simulink model "full_loop"  (R2020a)
settings: Solver=FixedStepAuto  StartTime=0.0  StopTime=200  FixedStep=.005  RelTol=1e-3
model workspace (MAT data in the model file):
  SL_ROS_VariableLengthArrays_MaxSizes.CommonInfo.ArrayTruncateAction = 'EmitWarning'
  SL_ROS_VariableLengthArrays_MaxSizes.MsgTypeMap = containers.Map
  SL_ROS_VariableLengthArrays_MaxSizes.MsgTypeMap.serialization.keys = {}
  SL_ROS_VariableLengthArrays_MaxSizes.MsgTypeMap.serialization.values = {}
  SL_ROS_VariableLengthArrays_MaxSizes.MsgTypeMap.serialization.uniformity = 0
  SL_ROS_VariableLengthArrays_MaxSizes.MsgTypeMap.serialization.keyType = 'char'
  SL_ROS_VariableLengthArrays_MaxSizes.MsgTypeMap.serialization.valueType = 'any'
undefined symbols (not defined in the file): cf, gazeboStep, InitAUVPlant, InitController, modelName, referenceFrame, telemetryStep, trajec
libraries: robotlib x8
settings Model: SimulationMode=accelerator  PauseTimes=1000  Creator=Lamarre  LastModifiedBy=alexemdesgagne
settings OptimizationCC: EnhancedBackFolding=on  PassReuseOutputArgsAs=Individual arguments  ZeroExternalMemoryAtStartup=off  ZeroInternalMemoryAtStartup=off  MaxStackSize=64  OptimizeBlockOrder=speed  DifferentSizesBufferReuse=on  OptimizationCustomize=off  EfficientTunableParamExpr=on
settings DebuggingCC: ParameterTunabilityLossMsg=error
settings HardwareCC: ProdBitPerPointer=32  ProdBitPerSizeT=32  ProdBitPerPtrDiffT=32  ProdLargestAtomicInteger=Long  ProdWordSize=32  ProdHWDeviceType=ARM Compatible->ARM 8
settings SFSimCC: MATLABDynamicMemAlloc=off
settings RTWCC: SystemTargetFile=ert.tlc  HardwareBoard=Robot Operating System (ROS)  TemplateMakefile=ert_default_tmf  Toolchain=Catkin  BuildConfiguration=Faster Runs  TargetLang=C++
settings CodeAppCC: ForceParamTrailComments=on  IgnoreCustomStorageClasses=off  OperatorAnnotations=on  SimulinkDataObjDesc=on  SFDataObjDesc=on  InsertBlockDesc=on
settings ERTTargetCC: MultiInstanceERTCode=on  CodeInterfacePackaging=C++ class  SupportContinuousTime=on  SupportVariableSizeSignals=on  RootIOFormat=Structure reference

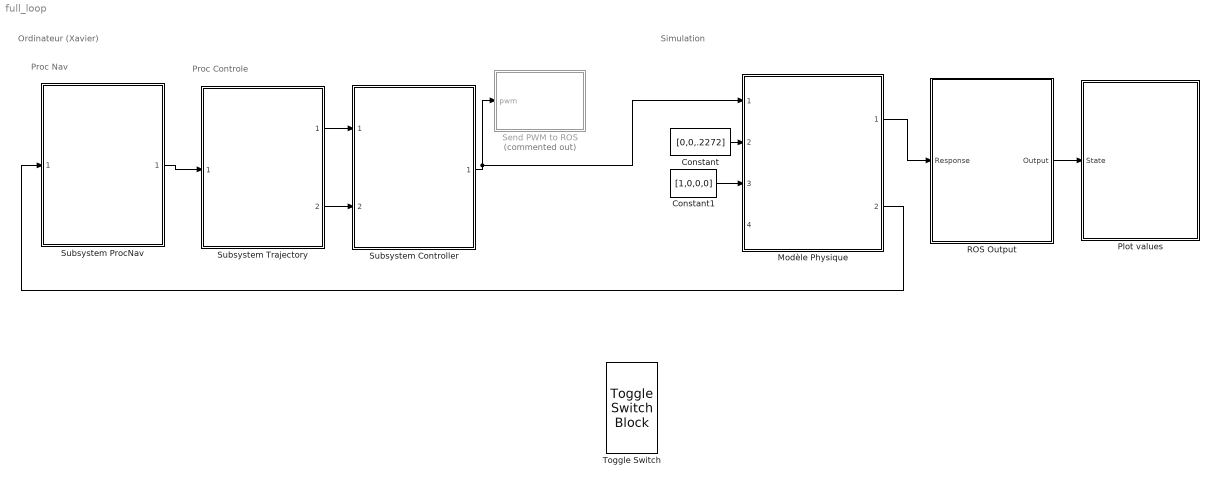
== system full_loop ==
  note: Simulation
  note: Proc Nav
  note: Proc Controle
  note: Ordinateur (Xavier)
  Constant : Constant  Value=[0,0,.2272]
  Constant1 : Constant  Value=[1,0,0,0]
  Modèle Physique : Subsystem  InitFcn=InitAUVPlant;  ReferencedSubsystem=AUVPlant
  Plot values : Subsystem
  ROS Output : Subsystem
  Send PWM to ROS : Subsystem  Commented=on
  Subsystem Controller : Subsystem  InitFcn=InitController;  ReferencedSubsystem=Controller
  Subsystem ProcNav : Subsystem  ReferencedSubsystem=ProcNav
  Subsystem Trajectory : Subsystem  InitFcn=trajec;  ReferencedSubsystem=Trajectory
  Toggle Switch : ToggleSwitchBlock
      settings: Values={{'Off', 'On'}, [0 1]}
  wires:
  Subsystem ProcNav/1 -> Subsystem Trajectory/1
  Subsystem Trajectory/1 -> Subsystem Controller/1
  Subsystem Controller/1 -> Modèle Physique/1, Send PWM to ROS/1(pwm)
  Modèle Physique/1 -> ROS Output/1(Response)
  Modèle Physique/2 -> Subsystem ProcNav/1
  Constant/1 -> Modèle Physique/2
  Constant1/1 -> Modèle Physique/3
  ROS Output/1(Output) -> Plot values/1(State)
  Subsystem Trajectory/2 -> Subsystem Controller/2

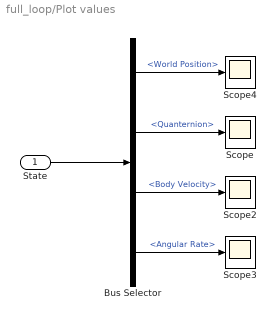
== system full_loop/Plot values ==
  State : Inport
  Bus Selector : BusSelector  OutputSignals=World Position,Quanternion,Body Velocity,Angular Rate
  Scope{,2..4} (4 alike) : Scope
  wires:
  Bus Selector/4 -> Scope3/1  "<Angular Rate>"
  State/1 -> Bus Selector/1
  Bus Selector/2 -> Scope/1  "<Quanternion>"
  Bus Selector/3 -> Scope2/1  "<Body Velocity>"
  Bus Selector/1 -> Scope4/1  "<World Position>"

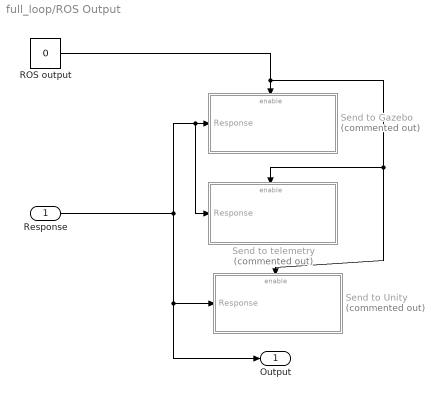
== system full_loop/ROS Output ==
  Response : Inport
  ROS output : Constant  Value=0
  Send to Gazebo : Subsystem  Commented=on  InitFcn=|
      | cf = ConfigAUV8();
      | 
      | % Parametres Messages ROS
      |     Duration = 229;
      |     gazeboStep=1/50;
      |     telemetryStep=1/30;
      |     referenceFrame = cf.referenceFrame;
      |     modelName = cf.modelName;
  Send to Unity : Subsystem  Commented=on  InitFcn=|
      | cf = ConfigAUV8();
      | 
      | % Parametres Messages ROS
      |     Duration = 229;
      |     gazeboStep=1/50;
      |     telemetryStep=1/30;
      |     referenceFrame = cf.referenceFrame;
      |     modelName = cf.modelName;
  Send to telemetry : Subsystem  Commented=on
  Output : Outport
  wires:
  Response/1 -> Send to telemetry/1(Response), Send to Gazebo/1(Response), Send to Unity/1(Response), Output/1
  ROS output/1 -> Send to Gazebo/Enable, Send to telemetry/Enable, Send to Unity/Enable

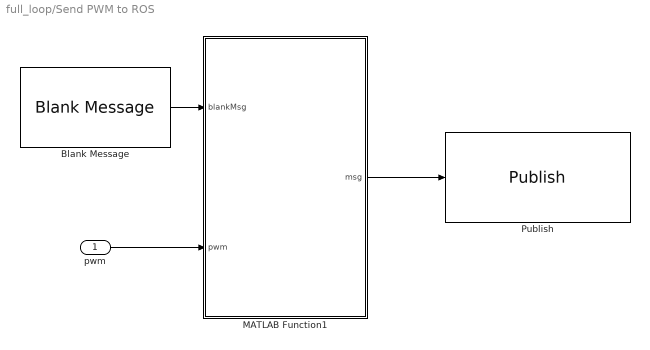
== system full_loop/Send PWM to ROS ==
  pwm : Inport
  Blank Message : robotlib/Blank Message  messageClass=Message  entityType=sonia_common/ThrusterPwm  messageType=sonia_common/ThrusterPwm  SampleTime=inf
  MATLAB Function1 : MATLAB Function  TreatAsAtomicUnit=on
  Publish : robotlib/Publish  topicSource=Specify your own  topic=/provider_thruster/thruster_pwm  messageType=sonia_common/ThrusterPwm  messageQueueLength=1
  wires:
  MATLAB Function1/1(msg) -> Publish/1
  Blank Message/1 -> MATLAB Function1/1(blankMsg)
  pwm/1 -> MATLAB Function1/2(pwm)

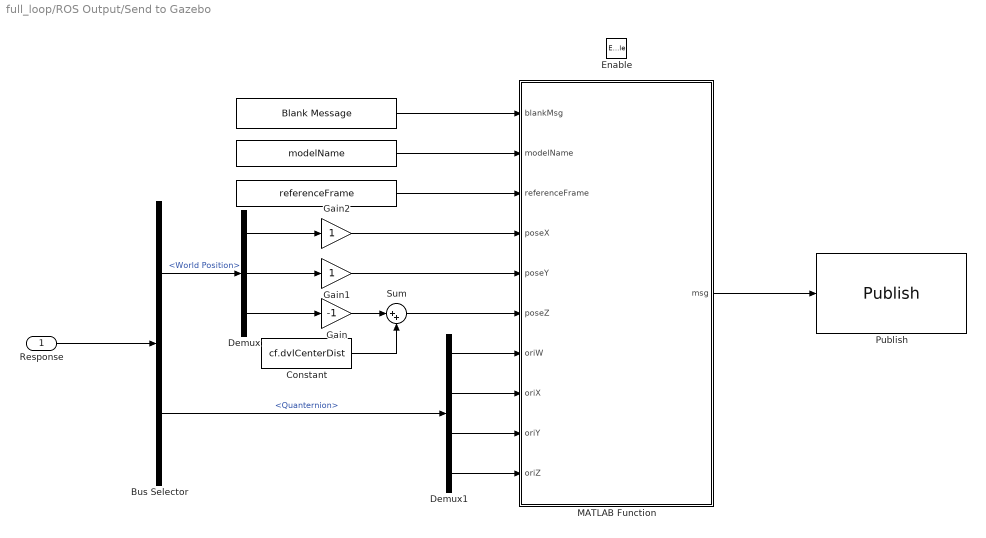
== system full_loop/ROS Output/Send to Gazebo ==
  Response : Inport
  Enable : EnablePort
  " " : Constant  Value=modelName  VectorParams1D=off
  "  " : Constant  Value=referenceFrame
  "   " : robotlib/Blank Message  messageClass=Message  entityType=gazebo_msgs/ModelState  messageType=gazebo_msgs/ModelState  SampleTime=1/50
  Bus Selector : BusSelector  OutputSignals=World Position,Quanternion
  Constant : Constant  Value=cf.dvlCenterDist
  Demux : Demux  Outputs=3
  Demux1 : Demux
  Gain : Gain  Gain=-1
  Gain1 : Gain
  Gain2 : Gain
  MATLAB Function : MATLAB Function  TreatAsAtomicUnit=on  SystemSampleTime=gazeboStep
  Publish : robotlib/Publish  topicSource=Select from ROS network  topic=/gazebo/set_model_state  messageType=gazebo_msgs/ModelState  messageQueueLength=1
      link override SinkBlock: ROSTopic=/gazebo/set_model_state  ROSMessageType=gazebo_msgs/ModelState  SLBusName=SL_Bus_plant_gazebo_msgs_ModelState  ModelName=plant  BlockId=Pub_plant_206
  Sum : Sum  Inputs=|++
  wires:
  Bus Selector/1 -> Demux/1  "<World Position>"
  Demux/1 -> Gain2/1
  Demux/2 -> Gain1/1
  Demux/3 -> Gain/1
  "   "/1 -> MATLAB Function/1(blankMsg)
  "  "/1 -> MATLAB Function/3(referenceFrame)
  " "/1 -> MATLAB Function/2(modelName)
  Gain1/1 -> MATLAB Function/5(poseY)
  Bus Selector/2 -> Demux1/1  "<Quanternion>"
  Demux1/1 -> MATLAB Function/7(oriW)
  Demux1/2 -> MATLAB Function/8(oriX)
  Demux1/3 -> MATLAB Function/9(oriY)
  Demux1/4 -> MATLAB Function/10(oriZ)
  Gain2/1 -> MATLAB Function/4(poseX)
  MATLAB Function/1(msg) -> Publish/1
  Response/1 -> Bus Selector/1
  Gain/1 -> Sum/1
  Sum/1 -> MATLAB Function/6(poseZ)
  Constant/1 -> Sum/2

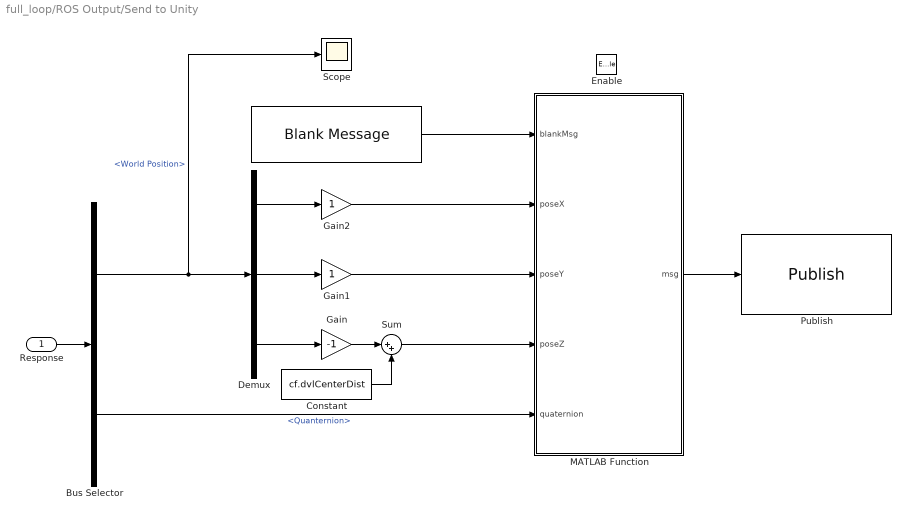
== system full_loop/ROS Output/Send to Unity ==
  Response : Inport
  Enable : EnablePort
  "   " : robotlib/Blank Message  messageClass=Message  entityType=auv_package/PosRot  messageType=auv_package/PosRot  SampleTime=1/50
  Bus Selector : BusSelector  OutputSignals=World Position,Quanternion
  Constant : Constant  Value=cf.dvlCenterDist
  Demux : Demux  Outputs=3
  Gain : Gain  Gain=-1
  Gain1 : Gain
  Gain2 : Gain
  MATLAB Function : MATLAB Function  TreatAsAtomicUnit=on  SystemSampleTime=gazeboStep
  Publish : robotlib/Publish  topicSource=Specify your own  topic=/pos_rot  messageType=auv_package/PosRot  messageQueueLength=1
      link override SinkBlock: ROSTopic=/gazebo/set_model_state  ROSMessageType=gazebo_msgs/ModelState  SLBusName=SL_Bus_plant_gazebo_msgs_ModelState  ModelName=plant  BlockId=Pub_plant_206
  Scope : Scope
  Sum : Sum  Inputs=|++
  wires:
  Bus Selector/1 -> Scope/1, Demux/1  "<World Position>"
  Demux/1 -> Gain2/1
  Demux/2 -> Gain1/1
  Demux/3 -> Gain/1
  "   "/1 -> MATLAB Function/1(blankMsg)
  Gain1/1 -> MATLAB Function/3(poseY)
  Bus Selector/2 -> MATLAB Function/5(quaternion)  "<Quanternion>"
  Gain2/1 -> MATLAB Function/2(poseX)
  MATLAB Function/1(msg) -> Publish/1
  Response/1 -> Bus Selector/1
  Gain/1 -> Sum/1
  Sum/1 -> MATLAB Function/4(poseZ)
  Constant/1 -> Sum/2

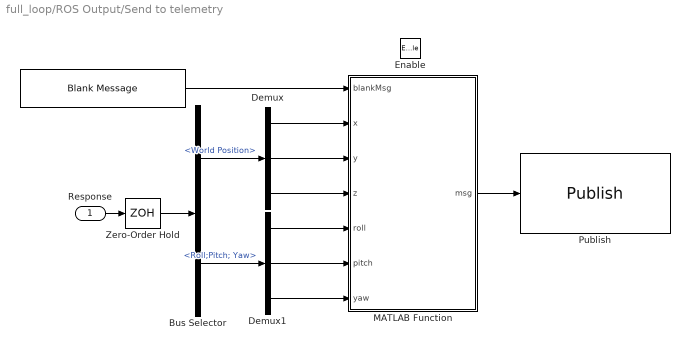
== system full_loop/ROS Output/Send to telemetry ==
  Response : Inport
  Enable : EnablePort
  "   " : robotlib/Blank Message  messageClass=Message  entityType=proc_control_matlab/Pose  messageType=proc_control_matlab/Pose  SampleTime=1/50
  Bus Selector : BusSelector  OutputSignals=World Position,Roll;Pitch; Yaw
  Demux : Demux  Outputs=3
  Demux1 : Demux  Outputs=3
  MATLAB Function : MATLAB Function  TreatAsAtomicUnit=on
  Publish : robotlib/Publish  topicSource=Specify your own  topic=/proc_control_matlab_Pose  messageType=proc_control_matlab/Pose  messageQueueLength=1
  Zero-Order Hold : ZeroOrderHold  SampleTime=telemetryStep
  wires:
  Demux/1 -> MATLAB Function/2(x)
  Demux1/2 -> MATLAB Function/6(pitch)
  Demux/3 -> MATLAB Function/4(z)
  Demux/2 -> MATLAB Function/3(y)
  Demux1/1 -> MATLAB Function/5(roll)
  MATLAB Function/1(msg) -> Publish/1
  Demux1/3 -> MATLAB Function/7(yaw)
  Bus Selector/2 -> Demux1/1  "<Roll;Pitch; Yaw>"
  Bus Selector/1 -> Demux/1  "<World Position>"
  Response/1 -> Zero-Order Hold/1
  "   "/1 -> MATLAB Function/1(blankMsg)
  Zero-Order Hold/1 -> Bus Selector/1

== matlab function full_loop/ROS Output/Send to Unity/MATLAB Function ==
  data: blankMsg input; poseX input; poseY input; poseZ input; msg output SL_Bus_full_loop_auv_package_pos_rot; quaternion input
function msg = assignUnityPoseRotInput(blankMsg, poseX, poseY, poseZ, quaternion)
% assignStringInput - Assign a string in a ROS message to specified input string
%
% MSG = assignStringInput(blankMsg, STR) assigns the input string, STR, to
%  a string field in the ROS message, blankMsg, and outputs the updated
%  ROS message.
%
%  Inputs
%    blankMsg: A bus for a 'std_msgs/String' message. This is 
%        used to initialize the output.
%    str: An array of uint8 that will be assigned to the 'Data' field
%        in blankMsg. The entire array is assumed to be a valid sequence of
%        character ASCII values.
% 
%  Outputs:
%    msg: A bus for a 'std_msgs/String' message, with the 'Data'
%        field set to a string.

%   Copyright 2015 The MathWorks, Inc.
%#codegen

% Note: The datatype of 'msg' has been explicitly set to the appropriate 
% Simulink bus type ("Bus: SL_Bus_robotROSMessageUsageExample_std_msgs_String"). 
%
% If the model name is changed, the datatype needs to be changed as well:
%   1) Click "Edit Data" in the Editor toolstrip to open "Ports and Data Manager"
%   2) Select "msg". From the "Type" dropdown, select "--- Refresh data types ---"
%   3) Set datatype to "Bus: SL_Bus_<modelname>_std_msgs_String"
   
msg = blankMsg;


msg.PosX = cast(poseX,'single');
msg.PosY = cast(poseY,'single');
msg.PosZ = cast(poseZ,'single');

msg.RotW = cast(quaternion(1),'single');
msg.RotX = cast(quaternion(2),'single');
msg.RotY = cast(quaternion(3),'single');
msg.RotZ = cast(quaternion(4),'single');

== matlab function full_loop/ROS Output/Send to Gazebo/MATLAB Function ==
  data: blankMsg input; msg output Bus: SL_Bus_full_loop_gazebo_msgs_ModelState; modelName input; referenceFrame input; poseX input; poseY input; poseZ input; oriW input; oriX input; oriY input; oriZ input
function msg = assignGazeboModelStateInput(blankMsg, modelName, referenceFrame, poseX, poseY, poseZ, oriW, oriX, oriY, oriZ)
% assignStringInput - Assign a string in a ROS message to specified input string
%
% MSG = assignStringInput(blankMsg, STR) assigns the input string, STR, to
%  a string field in the ROS message, blankMsg, and outputs the updated
%  ROS message.
%
%  Inputs
%    blankMsg: A bus for a 'std_msgs/String' message. This is 
%        used to initialize the output.
%    str: An array of uint8 that will be assigned to the 'Data' field
%        in blankMsg. The entire array is assumed to be a valid sequence of
%        character ASCII values.
% 
%  Outputs:
%    msg: A bus for a 'std_msgs/String' message, with the 'Data'
%        field set to a string.

%   Copyright 2015 The MathWorks, Inc.
%#codegen

% Note: The datatype of 'msg' has been explicitly set to the appropriate 
% Simulink bus type ("Bus: SL_Bus_robotROSMessageUsageExample_std_msgs_String"). 
%
% If the model name is changed, the datatype needs to be changed as well:
%   1) Click "Edit Data" in the Editor toolstrip to open "Ports and Data Manager"
%   2) Select "msg". From the "Type" dropdown, select "--- Refresh data types ---"
%   3) Set datatype to "Bus: SL_Bus_<modelname>_std_msgs_String"
   
msg = blankMsg;

strLength = length(modelName);
msg.ModelName(1:strLength) = modelName;
msg.ModelName_SL_Info.CurrentLength = uint32(strLength);

strLength = length(referenceFrame);
msg.ReferenceFrame(1:strLength) = referenceFrame;
msg.ReferenceFrame_SL_Info.CurrentLength = uint32(strLength);

msg.Pose.Position.X = poseX;
msg.Pose.Position.Y = poseY;
msg.Pose.Position.Z = poseZ;

msg.Pose.Orientation.X = oriX;
msg.Pose.Orientation.Y = oriY;
msg.Pose.Orientation.Z = oriZ;
msg.Pose.Orientation.W = oriW;

== matlab function full_loop/Send PWM to ROS/MATLAB Function1 ==
  data: blankMsg input; pwm input; msg output Bus: SL_Bus_full_loop_sonia_common_ThrusterPwm
function msg = assignThrusterPwm(blankMsg, pwm)
msg = blankMsg;
msg.Pwm(1:8) = cast(pwm, 'uint16');
msg.Pwm_SL_Info.CurrentLength = uint32(8);

== matlab function full_loop/ROS Output/Send to telemetry/MATLAB Function ==
  data: blankMsg input; x input; msg output Bus: SL_Bus_plant_proc_control_matlab_Pose; y input; z input; roll input; pitch input; yaw input
function msg = assignPoseInput(blankMsg, x, y, z, roll, pitch, yaw)
msg = blankMsg;
msg.X = x;
msg.Y = y;
msg.Z = z;
msg.Roll = roll;
msg.Pitch = pitch;
msg.Yaw = yaw;
